simulink model "MotorBlokdiagram"  (R2020b)
settings: Solver=VariableStepAuto  StartTime=0.0  StopTime=10.0  RelTol=1e-3
model workspace (MAT data in the model file):
  E_a = 5
  L_m = 1
  R_m = 1
  V_ref = 1
settings Model: Creator=henri  LastModifiedBy=jonas

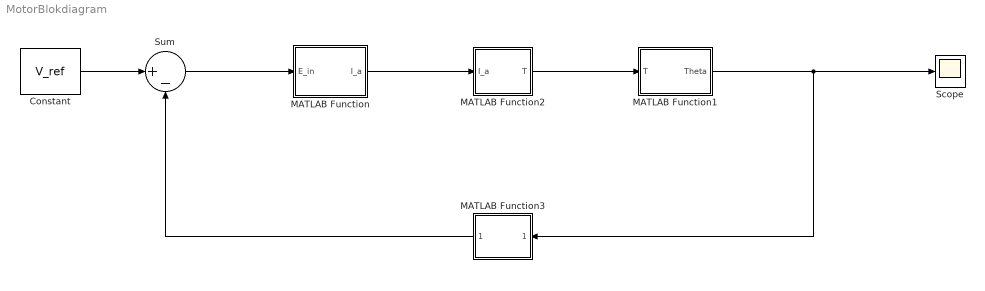
== system MotorBlokdiagram ==
  Constant : Constant  Value=V_ref
      mask Display: image('C:\Users\jonas\Desktop\Vref.png'); % Use "Edit Image" on toolstrip to change.
  MATLAB Function : MATLAB Function  TreatAsAtomicUnit=on
  MATLAB Function1 : MATLAB Function  TreatAsAtomicUnit=on
  MATLAB Function2 : MATLAB Function  TreatAsAtomicUnit=on
  MATLAB Function3 : MATLAB Function  TreatAsAtomicUnit=on
  Scope : Scope
  Sum : Sum  Inputs=|+-
  wires:
  Constant/1 -> Sum/1
  Sum/1 -> MATLAB Function/1(E_in)
  MATLAB Function/1(I_a) -> MATLAB Function2/1(I_a)
  MATLAB Function2/1(T) -> MATLAB Function1/1(T)
  MATLAB Function1/1(Theta) -> MATLAB Function3/1(Theta), Scope/1
  MATLAB Function3/1(Error) -> Sum/2

== matlab function MotorBlokdiagram/MATLAB Function ==
  data: E_in input; I_a output
function I_a = fcn(E_in)

I_a = 1/(s*L_m + R_m)

== matlab function MotorBlokdiagram/MATLAB Function2 ==
  data: I_a input; T output
function T = fcn(I_a)

T=K_t*I_a;

== matlab function MotorBlokdiagram/MATLAB Function3 ==
  data: Theta input; Error output
function Error = fcn(Theta)
Error = K_m *s *Theta;

== matlab function MotorBlokdiagram/MATLAB Function1 ==
  data: T input; Theta output
function Theta = fcn(T)
Theta= 1/(J*s^2 + B*s);
